simulink model "Relu_OutFB_4_4_1_HW_C6"  (R2012b)
settings: Solver=ode45  StartTime=0.0  StopTime=10.0  RelTol=1e-3
undefined symbols (not defined in the file): alpha, delayMulx, delayMuly, delayROMSig, M2, M3, mu, ts
libraries: xbsIndex_r4 x1583, roblocks x1
(part 3 of 13)

== system Relu_OutFB_4_4_1_HW_C6/EN_MLP_BK_(1,4_NL,1_L)_HW_FPGA/MLP_BK_(2,4_NL,1_L)_HW_FPGA/BK (2,4_NL,1_L)/Subsystem1 ==
  z_1(n) : Inport
  Wy_11(n) : Inport  Port=2
  Gy_11(n) : Inport  Port=3
  Constant : xbsIndex_r4/Constant  const=0  gui_display_data_type=Fixed-point  arith_type=Signed (2's comp)  n_bits=nb  bin_pt=bp  preci_type=Single  exp_width=8  frac_width=24  explicit_period=off  period=1  equ=P=C  opselect=C  inp2=PCIN>>17  opr=+  inp1=P  carry=CIN  dbl_ovrd=off  block_type=constant
  Reinterpret : xbsIndex_r4/Reinterpret  force_arith_type=on  arith_type="Signed  (2's comp)"  force_bin_pt=on  bin_pt=0  block_type=reinterpret
  Relational : xbsIndex_r4/Relational  mode=a<=b  en=off  latency=0  dbl_ovrd=off  block_type=relational
  w_ij(n)*Gy(n) : xbsIndex_r4/Mult  precision=User Defined  arith_type="Signed  (2's comp)"  n_bits=nb  bin_pt=bp  quantization="Round  (unbiased: +/- Inf)"  overflow=Saturate  en=off  latency=delayMuly  dbl_ovrd=off  use_behavioral_HDL=off  opt=Speed  use_embedded=on  optimum_pipeline=off  pipeline=on  use_rpm=on  placement_style=Triangular  block_type=mult
  w_ij(n)*Gy(n)1 : xbsIndex_r4/Mult  precision=User Defined  arith_type="Signed  (2's comp)"  n_bits=nb  bin_pt=bp  quantization="Round  (unbiased: +/- Inf)"  overflow=Saturate  en=off  latency=delayMuly  dbl_ovrd=off  use_behavioral_HDL=off  opt=Speed  use_embedded=on  optimum_pipeline=off  pipeline=on  use_rpm=on  placement_style=Triangular  block_type=mult
  Gx_1(n) : Outport
  wires:
  w_ij(n)*Gy(n)1/1 -> Gx_1(n)/1
  Relational/1 -> Reinterpret/1
  Gy_11(n)/1 -> w_ij(n)*Gy(n)/2
  w_ij(n)*Gy(n)/1 -> w_ij(n)*Gy(n)1/2
  Wy_11(n)/1 -> w_ij(n)*Gy(n)/1
  Constant/1 -> Relational/2
  z_1(n)/1 -> Relational/1
  Reinterpret/1 -> w_ij(n)*Gy(n)1/1

== system Relu_OutFB_4_4_1_HW_C6/EN_MLP_BK_(1,4_NL,1_L)_HW_FPGA/MLP_BK_(2,4_NL,1_L)_HW_FPGA/BK (2,4_NL,1_L)/Subsystem2 ==
  x_0(n) : Inport
  x_1(n) : Inport  Port=2
  Gx_1(n) : Inport  Port=3
  x_2(n) : Inport  Port=4
  x_3(n) : Inport  Port=5
  x_4(n) : Inport  Port=6
  Subsystem1 : Subsystem
  Subsystem2 : Subsystem
  Subsystem3 : Subsystem
  Subsystem5 : Subsystem
  Subsystem6 : Subsystem
  Wx_21(n) : Outport
  Wx_20(n) : Outport  Port=2
  Wx_22(n) : Outport  Port=3
  Wx_23(n) : Outport  Port=4
  Wx_24(n) : Outport  Port=5
  wires:
  Subsystem3/1(Wx_11(n)) -> Wx_24(n)/1
  x_4(n)/1 -> Subsystem3/2(x_1(n))
  Gx_1(n)/1 -> Subsystem6/1(Gx_1(n)), Subsystem1/1(Gx_1(n)), Subsystem2/1(Gx_1(n)), Subsystem3/1(Gx_1(n)), Subsystem5/1(Gx_1(n))
  Subsystem1/1(Wx_11(n)) -> Wx_22(n)/1
  Subsystem2/1(Wx_11(n)) -> Wx_23(n)/1
  x_2(n)/1 -> Subsystem1/2(x_1(n))
  x_3(n)/1 -> Subsystem2/2(x_1(n))
  x_1(n)/1 -> Subsystem6/2(x_1(n))
  Subsystem6/1(Wx_11(n)) -> Wx_21(n)/1
  x_0(n)/1 -> Subsystem5/2(x_0(n))
  Subsystem5/1(Wx_10(n)) -> Wx_20(n)/1

== system Relu_OutFB_4_4_1_HW_C6/EN_MLP_BK_(1,4_NL,1_L)_HW_FPGA/MLP_BK_(2,4_NL,1_L)_HW_FPGA/BK (2,4_NL,1_L)/Subsystem3 ==
  z_1(n) : Inport
  Wy_11(n) : Inport  Port=2
  Gy_11(n) : Inport  Port=3
  Constant : xbsIndex_r4/Constant  const=0  gui_display_data_type=Fixed-point  arith_type=Signed (2's comp)  n_bits=nb  bin_pt=bp  preci_type=Single  exp_width=8  frac_width=24  explicit_period=off  period=1  equ=P=C  opselect=C  inp2=PCIN>>17  opr=+  inp1=P  carry=CIN  dbl_ovrd=off  block_type=constant
  Reinterpret : xbsIndex_r4/Reinterpret  force_arith_type=on  arith_type="Signed  (2's comp)"  force_bin_pt=on  bin_pt=0  block_type=reinterpret
  Relational : xbsIndex_r4/Relational  mode=a<=b  en=off  latency=0  dbl_ovrd=off  block_type=relational
  w_ij(n)*Gy(n) : xbsIndex_r4/Mult  precision=User Defined  arith_type="Signed  (2's comp)"  n_bits=nb  bin_pt=bp  quantization="Round  (unbiased: +/- Inf)"  overflow=Saturate  en=off  latency=delayMuly  dbl_ovrd=off  use_behavioral_HDL=off  opt=Speed  use_embedded=on  optimum_pipeline=off  pipeline=on  use_rpm=on  placement_style=Triangular  block_type=mult
  w_ij(n)*Gy(n)1 : xbsIndex_r4/Mult  precision=User Defined  arith_type="Signed  (2's comp)"  n_bits=nb  bin_pt=bp  quantization="Round  (unbiased: +/- Inf)"  overflow=Saturate  en=off  latency=delayMuly  dbl_ovrd=off  use_behavioral_HDL=off  opt=Speed  use_embedded=on  optimum_pipeline=off  pipeline=on  use_rpm=on  placement_style=Triangular  block_type=mult
  Gx_1(n) : Outport
  wires:
  w_ij(n)*Gy(n)1/1 -> Gx_1(n)/1
  Relational/1 -> Reinterpret/1
  Gy_11(n)/1 -> w_ij(n)*Gy(n)/2
  w_ij(n)*Gy(n)/1 -> w_ij(n)*Gy(n)1/2
  Wy_11(n)/1 -> w_ij(n)*Gy(n)/1
  Constant/1 -> Relational/2
  z_1(n)/1 -> Relational/1
  Reinterpret/1 -> w_ij(n)*Gy(n)1/1

== system Relu_OutFB_4_4_1_HW_C6/EN_MLP_BK_(1,4_NL,1_L)_HW_FPGA/MLP_BK_(2,4_NL,1_L)_HW_FPGA/BK (2,4_NL,1_L)/Subsystem4 ==
  z_1(n) : Inport
  Wy_11(n) : Inport  Port=2
  Gy_11(n) : Inport  Port=3
  Constant : xbsIndex_r4/Constant  const=0  gui_display_data_type=Fixed-point  arith_type=Signed (2's comp)  n_bits=nb  bin_pt=bp  preci_type=Single  exp_width=8  frac_width=24  explicit_period=off  period=1  equ=P=C  opselect=C  inp2=PCIN>>17  opr=+  inp1=P  carry=CIN  dbl_ovrd=off  block_type=constant
  Reinterpret : xbsIndex_r4/Reinterpret  force_arith_type=on  arith_type="Signed  (2's comp)"  force_bin_pt=on  bin_pt=0  block_type=reinterpret
  Relational : xbsIndex_r4/Relational  mode=a<=b  en=off  latency=0  dbl_ovrd=off  block_type=relational
  w_ij(n)*Gy(n) : xbsIndex_r4/Mult  precision=User Defined  arith_type="Signed  (2's comp)"  n_bits=nb  bin_pt=bp  quantization="Round  (unbiased: +/- Inf)"  overflow=Saturate  en=off  latency=delayMuly  dbl_ovrd=off  use_behavioral_HDL=off  opt=Speed  use_embedded=on  optimum_pipeline=off  pipeline=on  use_rpm=on  placement_style=Triangular  block_type=mult
  w_ij(n)*Gy(n)1 : xbsIndex_r4/Mult  precision=User Defined  arith_type="Signed  (2's comp)"  n_bits=nb  bin_pt=bp  quantization="Round  (unbiased: +/- Inf)"  overflow=Saturate  en=off  latency=delayMuly  dbl_ovrd=off  use_behavioral_HDL=off  opt=Speed  use_embedded=on  optimum_pipeline=off  pipeline=on  use_rpm=on  placement_style=Triangular  block_type=mult
  Gx_1(n) : Outport
  wires:
  w_ij(n)*Gy(n)1/1 -> Gx_1(n)/1
  Relational/1 -> Reinterpret/1
  Gy_11(n)/1 -> w_ij(n)*Gy(n)/2
  w_ij(n)*Gy(n)/1 -> w_ij(n)*Gy(n)1/2
  Wy_11(n)/1 -> w_ij(n)*Gy(n)/1
  Constant/1 -> Relational/2
  z_1(n)/1 -> Relational/1
  Reinterpret/1 -> w_ij(n)*Gy(n)1/1

== system Relu_OutFB_4_4_1_HW_C6/EN_MLP_BK_(1,4_NL,1_L)_HW_FPGA/MLP_BK_(2,4_NL,1_L)_HW_FPGA/BK (2,4_NL,1_L)/Subsystem5 ==
  x_0(n) : Inport
  x_1(n) : Inport  Port=2
  Gx_1(n) : Inport  Port=3
  x_2(n) : Inport  Port=4
  x_3(n) : Inport  Port=5
  x_4(n) : Inport  Port=6
  Subsystem1 : Subsystem
  Subsystem2 : Subsystem
  Subsystem3 : Subsystem
  Subsystem5 : Subsystem
  Subsystem6 : Subsystem
  Wx_31(n) : Outport
  Wx_30(n) : Outport  Port=2
  Wx_32(n) : Outport  Port=3
  Wx_33(n) : Outport  Port=4
  Wx_34(n) : Outport  Port=5
  wires:
  Subsystem5/1(Wx_10(n)) -> Wx_30(n)/1
  x_0(n)/1 -> Subsystem5/2(x_0(n))
  Subsystem6/1(Wx_11(n)) -> Wx_31(n)/1
  x_1(n)/1 -> Subsystem6/2(x_1(n))
  x_3(n)/1 -> Subsystem2/2(x_1(n))
  x_2(n)/1 -> Subsystem1/2(x_1(n))
  Subsystem2/1(Wx_11(n)) -> Wx_33(n)/1
  Subsystem1/1(Wx_11(n)) -> Wx_32(n)/1
  Gx_1(n)/1 -> Subsystem5/1(Gx_1(n)), Subsystem3/1(Gx_1(n)), Subsystem2/1(Gx_1(n)), Subsystem1/1(Gx_1(n)), Subsystem6/1(Gx_1(n))
  x_4(n)/1 -> Subsystem3/2(x_1(n))
  Subsystem3/1(Wx_11(n)) -> Wx_34(n)/1

== system Relu_OutFB_4_4_1_HW_C6/EN_MLP_BK_(1,4_NL,1_L)_HW_FPGA/MLP_BK_(2,4_NL,1_L)_HW_FPGA/BK (2,4_NL,1_L)/Subsystem6 ==
  x_0(n) : Inport
  x_1(n) : Inport  Port=2
  Gx_1(n) : Inport  Port=3
  x_2(n) : Inport  Port=4
  x_3(n) : Inport  Port=5
  x_4(n) : Inport  Port=6
  Subsystem1 : Subsystem
  Subsystem2 : Subsystem
  Subsystem3 : Subsystem
  Subsystem5 : Subsystem
  Subsystem6 : Subsystem
  Wx_41(n) : Outport
  Wx_40(n) : Outport  Port=2
  Wx_42(n) : Outport  Port=3
  Wx_43(n) : Outport  Port=4
  Wx_44(n) : Outport  Port=5
  wires:
  Subsystem3/1(Wx_11(n)) -> Wx_44(n)/1
  x_4(n)/1 -> Subsystem3/2(x_1(n))
  Gx_1(n)/1 -> Subsystem6/1(Gx_1(n)), Subsystem1/1(Gx_1(n)), Subsystem2/1(Gx_1(n)), Subsystem3/1(Gx_1(n)), Subsystem5/1(Gx_1(n))
  Subsystem1/1(Wx_11(n)) -> Wx_42(n)/1
  Subsystem2/1(Wx_11(n)) -> Wx_43(n)/1
  x_2(n)/1 -> Subsystem1/2(x_1(n))
  x_3(n)/1 -> Subsystem2/2(x_1(n))
  x_1(n)/1 -> Subsystem6/2(x_1(n))
  Subsystem6/1(Wx_11(n)) -> Wx_41(n)/1
  x_0(n)/1 -> Subsystem5/2(x_0(n))
  Subsystem5/1(Wx_10(n)) -> Wx_40(n)/1

== system Relu_OutFB_4_4_1_HW_C6/EN_MLP_BK_(1,4_NL,1_L)_HW_FPGA/MLP_BK_(2,4_NL,1_L)_HW_FPGA/BK (2,4_NL,1_L)/Subsystem7 ==
  z_1(n) : Inport
  Wy_11(n) : Inport  Port=2
  Gy_11(n) : Inport  Port=3
  Constant : xbsIndex_r4/Constant  const=0  gui_display_data_type=Fixed-point  arith_type=Signed (2's comp)  n_bits=nb  bin_pt=bp  preci_type=Single  exp_width=8  frac_width=24  explicit_period=off  period=1  equ=P=C  opselect=C  inp2=PCIN>>17  opr=+  inp1=P  carry=CIN  dbl_ovrd=off  block_type=constant
  Reinterpret : xbsIndex_r4/Reinterpret  force_arith_type=on  arith_type="Signed  (2's comp)"  force_bin_pt=on  bin_pt=0  block_type=reinterpret
  Relational : xbsIndex_r4/Relational  mode=a<=b  en=off  latency=0  dbl_ovrd=off  block_type=relational
  w_ij(n)*Gy(n) : xbsIndex_r4/Mult  precision=User Defined  arith_type="Signed  (2's comp)"  n_bits=nb  bin_pt=bp  quantization="Round  (unbiased: +/- Inf)"  overflow=Saturate  en=off  latency=delayMuly  dbl_ovrd=off  use_behavioral_HDL=off  opt=Speed  use_embedded=on  optimum_pipeline=off  pipeline=on  use_rpm=on  placement_style=Triangular  block_type=mult
  w_ij(n)*Gy(n)1 : xbsIndex_r4/Mult  precision=User Defined  arith_type="Signed  (2's comp)"  n_bits=nb  bin_pt=bp  quantization="Round  (unbiased: +/- Inf)"  overflow=Saturate  en=off  latency=delayMuly  dbl_ovrd=off  use_behavioral_HDL=off  opt=Speed  use_embedded=on  optimum_pipeline=off  pipeline=on  use_rpm=on  placement_style=Triangular  block_type=mult
  Gx_1(n) : Outport
  wires:
  w_ij(n)*Gy(n)1/1 -> Gx_1(n)/1
  Relational/1 -> Reinterpret/1
  Gy_11(n)/1 -> w_ij(n)*Gy(n)/2
  w_ij(n)*Gy(n)/1 -> w_ij(n)*Gy(n)1/2
  Wy_11(n)/1 -> w_ij(n)*Gy(n)/1
  Constant/1 -> Relational/2
  z_1(n)/1 -> Relational/1
  Reinterpret/1 -> w_ij(n)*Gy(n)1/1

== system Relu_OutFB_4_4_1_HW_C6/EN_MLP_BK_(1,4_NL,1_L)_HW_FPGA/MLP_BK_(2,4_NL,1_L)_HW_FPGA/BK (2,4_NL,1_L)/Subsystem8 ==
  x_0(n) : Inport
  x_1(n) : Inport  Port=2
  Gx_1(n) : Inport  Port=3
  x_2(n) : Inport  Port=4
  x_3(n) : Inport  Port=5
  x_4(n) : Inport  Port=6
  Subsystem1 : Subsystem
  Subsystem2 : Subsystem
  Subsystem3 : Subsystem
  Subsystem5 : Subsystem
  Subsystem6 : Subsystem
  Wx_11(n) : Outport
  Wx_10(n) : Outport  Port=2
  Wx_12(n) : Outport  Port=3
  Wx_13(n) : Outport  Port=4
  Wx_14(n) : Outport  Port=5
  wires:
  Subsystem5/1(Wx_10(n)) -> Wx_10(n)/1
  x_0(n)/1 -> Subsystem5/2(x_0(n))
  Subsystem6/1(Wx_11(n)) -> Wx_11(n)/1
  x_1(n)/1 -> Subsystem6/2(x_1(n))
  x_3(n)/1 -> Subsystem2/2(x_1(n))
  x_2(n)/1 -> Subsystem1/2(x_1(n))
  Subsystem2/1(Wx_13(n)) -> Wx_13(n)/1
  Subsystem1/1(Wx_12(n)) -> Wx_12(n)/1
  Gx_1(n)/1 -> Subsystem5/1(Gx_1(n)), Subsystem3/1(Gx_1(n)), Subsystem2/1(Gx_1(n)), Subsystem1/1(Gx_1(n)), Subsystem6/1(Gx_1(n))
  x_4(n)/1 -> Subsystem3/2(x_1(n))
  Subsystem3/1(Wx_14(n)) -> Wx_14(n)/1

== system Relu_OutFB_4_4_1_HW_C6/EN_MLP_BK_(1,4_NL,1_L)_HW_FPGA/MLP_BK_(2,4_NL,1_L)_HW_FPGA/MLP (2,4_NL,1_L)/Neurônio Linear_HW2 ==
  note: x_p
  note: x_p
  note: x_p
  note: x_p
  note: x_p
  z_0(n) : Inport
  z_1(n) : Inport  Port=2
  z_2(n)1 : Inport  Port=3
  z_3(n)2 : Inport  Port=4
  z_4(n)3 : Inport  Port=5
  w_ij(n)4 : Inport  Port=6
  w_ij(n) : Inport  Port=7
  w_ij(n)1 : Inport  Port=8
  w_ij(n)2 : Inport  Port=9
  w_ij(n)3 : Inport  Port=10
  AddSub{,1..3} (4 alike) : xbsIndex_r4/AddSub  mode=Addition  use_carryin=off  use_carryout=off  en=off  latency=0  precision=User Defined  arith_type="Signed  (2's comp)"  n_bits=nb  bin_pt=bp  quantization="Round  (unbiased: +/- Inf)"  overflow=Wrap  dbl_ovrd=off  use_behavioral_HDL=off  hw_selection=Fabric  pipelined=off  block_type=addsub
  x_p*w_ij(n){,1..4} (5 alike) : xbsIndex_r4/Mult  precision=User Defined  arith_type="Signed  (2's comp)"  n_bits=nb  bin_pt=bp  quantization="Round  (unbiased: +/- Inf)"  overflow=Saturate  en=off  latency=delayMuly  dbl_ovrd=off  use_behavioral_HDL=off  opt=Speed  use_embedded=on  optimum_pipeline=off  pipeline=on  use_rpm=on  placement_style=Triangular  block_type=mult
  y_0(n) : Outport
  wires:
  AddSub2/1 -> AddSub3/2
  w_ij(n)4/1 -> x_p*w_ij(n)4/1  "w_ij(n)"
  z_0(n)/1 -> x_p*w_ij(n)4/2
  x_p*w_ij(n)4/1 -> AddSub3/1  "y_k"
  AddSub1/1 -> AddSub2/2
  AddSub/1 -> AddSub2/1
  w_ij(n)2/1 -> x_p*w_ij(n)2/1  "w_ij(n)"
  z_3(n)2/1 -> x_p*w_ij(n)2/2
  x_p*w_ij(n)2/1 -> AddSub1/1  "y_k"
  w_ij(n)3/1 -> x_p*w_ij(n)3/1  "w_ij(n)"
  z_4(n)3/1 -> x_p*w_ij(n)3/2
  x_p*w_ij(n)3/1 -> AddSub1/2
  w_ij(n)/1 -> x_p*w_ij(n)/1  "w_ij(n)"
  z_1(n)/1 -> x_p*w_ij(n)/2
  x_p*w_ij(n)/1 -> AddSub/1  "y_k"
  w_ij(n)1/1 -> x_p*w_ij(n)1/1  "w_ij(n)"
  z_2(n)1/1 -> x_p*w_ij(n)1/2
  x_p*w_ij(n)1/1 -> AddSub/2
  AddSub3/1 -> y_0(n)/1

== system Relu_OutFB_4_4_1_HW_C6/EN_MLP_BK_(1,4_NL,1_L)_HW_FPGA/MLP_BK_(2,4_NL,1_L)_HW_FPGA/MLP (2,4_NL,1_L)/Neurônio Não-Linear_HW1 ==
  note: x_p
  note: x_p
  x_0(n) : Inport
  x_1(n) : Inport  Port=2
  x_2(n) : Inport  Port=3
  x_3(n) : Inport  Port=4
  x_4(n) : Inport  Port=5
  Wx_20(n) : Inport  Port=6
  Wx_21(n) : Inport  Port=7
  Wx_22(n) : Inport  Port=8
  Wx_23(n) : Inport  Port=9
  Wx_24(n) : Inport  Port=10
  AddSub{1..4} (4 alike) : xbsIndex_r4/AddSub  mode=Addition  use_carryin=off  use_carryout=off  en=off  latency=0  precision=User Defined  arith_type="Signed  (2's comp)"  n_bits=nb  bin_pt=bp  quantization="Round  (unbiased: +/- Inf)"  overflow=Wrap  dbl_ovrd=off  use_behavioral_HDL=off  hw_selection=Fabric  pipelined=off  block_type=addsub
  Subsystem : Subsystem
  x_p*w_ij(n){,1..4} (5 alike) : xbsIndex_r4/Mult  precision=User Defined  arith_type="Signed  (2's comp)"  n_bits=nb  bin_pt=bp  quantization="Round  (unbiased: +/- Inf)"  overflow=Saturate  en=off  latency=delayMulx  dbl_ovrd=off  use_behavioral_HDL=off  opt=Speed  use_embedded=on  optimum_pipeline=off  pipeline=on  use_rpm=on  placement_style=Triangular  block_type=mult
  z_k(n) : Outport
  wires:
  Wx_21(n)/1 -> x_p*w_ij(n)/1  "w_ij(n)"
  x_1(n)/1 -> x_p*w_ij(n)/2
  x_p*w_ij(n)/1 -> AddSub1/2  "y_k"
  Subsystem/1(Out1) -> z_k(n)/1
  Wx_20(n)/1 -> x_p*w_ij(n)2/1  "w_ij(n)"
  x_0(n)/1 -> x_p*w_ij(n)2/2
  x_p*w_ij(n)2/1 -> AddSub1/1
  x_2(n)/1 -> x_p*w_ij(n)1/2
  x_3(n)/1 -> x_p*w_ij(n)3/2
  x_4(n)/1 -> x_p*w_ij(n)4/2
  Wx_22(n)/1 -> x_p*w_ij(n)1/1
  Wx_23(n)/1 -> x_p*w_ij(n)3/1
  Wx_24(n)/1 -> x_p*w_ij(n)4/1
  x_p*w_ij(n)1/1 -> AddSub2/1
  x_p*w_ij(n)3/1 -> AddSub2/2
  x_p*w_ij(n)4/1 -> AddSub3/2
  AddSub2/1 -> AddSub3/1
  AddSub4/1 -> Subsystem/1(In1)
  AddSub3/1 -> AddSub4/2
  AddSub1/1 -> AddSub4/1

== system Relu_OutFB_4_4_1_HW_C6/EN_MLP_BK_(1,4_NL,1_L)_HW_FPGA/MLP_BK_(2,4_NL,1_L)_HW_FPGA/MLP (2,4_NL,1_L)/Neurônio Não-Linear_HW2 ==
  note: x_p
  note: x_p
  x_0(n) : Inport
  x_1(n) : Inport  Port=2
  x_2(n) : Inport  Port=3
  x_3(n) : Inport  Port=4
  x_4(n) : Inport  Port=5
  Wx_10(n) : Inport  Port=6
  Wx_11(n) : Inport  Port=7
  Wx_12(n) : Inport  Port=8
  Wx_13(n) : Inport  Port=9
  Wx_14(n) : Inport  Port=10
  AddSub{1..4} (4 alike) : xbsIndex_r4/AddSub  mode=Addition  use_carryin=off  use_carryout=off  en=off  latency=0  precision=User Defined  arith_type="Signed  (2's comp)"  n_bits=nb  bin_pt=bp  quantization="Round  (unbiased: +/- Inf)"  overflow=Wrap  dbl_ovrd=off  use_behavioral_HDL=off  hw_selection=Fabric  pipelined=off  block_type=addsub
  Subsystem : Subsystem
  x_p*w_ij(n){,1..4} (5 alike) : xbsIndex_r4/Mult  precision=User Defined  arith_type="Signed  (2's comp)"  n_bits=nb  bin_pt=bp  quantization="Round  (unbiased: +/- Inf)"  overflow=Saturate  en=off  latency=delayMulx  dbl_ovrd=off  use_behavioral_HDL=off  opt=Speed  use_embedded=on  optimum_pipeline=off  pipeline=on  use_rpm=on  placement_style=Triangular  block_type=mult
  z_k(n) : Outport
  wires:
  AddSub1/1 -> AddSub4/1
  AddSub4/1 -> Subsystem/1(In1)
  AddSub2/1 -> AddSub3/1
  x_p*w_ij(n)4/1 -> AddSub3/2
  x_p*w_ij(n)3/1 -> AddSub2/2
  x_p*w_ij(n)1/1 -> AddSub2/1
  Wx_14(n)/1 -> x_p*w_ij(n)4/1
  Wx_13(n)/1 -> x_p*w_ij(n)3/1
  Wx_12(n)/1 -> x_p*w_ij(n)1/1
  x_4(n)/1 -> x_p*w_ij(n)4/2
  x_3(n)/1 -> x_p*w_ij(n)3/2
  x_2(n)/1 -> x_p*w_ij(n)1/2
  x_p*w_ij(n)2/1 -> AddSub1/1
  x_0(n)/1 -> x_p*w_ij(n)2/2
  Wx_10(n)/1 -> x_p*w_ij(n)2/1  "w_ij(n)"
  Subsystem/1(Out1) -> z_k(n)/1
  x_p*w_ij(n)/1 -> AddSub1/2  "y_k"
  x_1(n)/1 -> x_p*w_ij(n)/2
  Wx_11(n)/1 -> x_p*w_ij(n)/1  "w_ij(n)"
  AddSub3/1 -> AddSub4/2

== system Relu_OutFB_4_4_1_HW_C6/EN_MLP_BK_(1,4_NL,1_L)_HW_FPGA/MLP_BK_(2,4_NL,1_L)_HW_FPGA/MLP (2,4_NL,1_L)/Neurônio Não-Linear_HW3 ==
  note: x_p
  note: x_p
  x_0(n) : Inport
  x_1(n) : Inport  Port=2
  x_2(n) : Inport  Port=3
  x_3(n) : Inport  Port=4
  x_4(n) : Inport  Port=5
  Wx_30(n) : Inport  Port=6
  Wx_31(n) : Inport  Port=7
  Wx_32(n) : Inport  Port=8
  Wx_33(n) : Inport  Port=9
  Wx_34(n) : Inport  Port=10
  AddSub{1..4} (4 alike) : xbsIndex_r4/AddSub  mode=Addition  use_carryin=off  use_carryout=off  en=off  latency=0  precision=User Defined  arith_type="Signed  (2's comp)"  n_bits=nb  bin_pt=bp  quantization="Round  (unbiased: +/- Inf)"  overflow=Wrap  dbl_ovrd=off  use_behavioral_HDL=off  hw_selection=Fabric  pipelined=off  block_type=addsub
  Subsystem : Subsystem
  x_p*w_ij(n){,1..4} (5 alike) : xbsIndex_r4/Mult  precision=User Defined  arith_type="Signed  (2's comp)"  n_bits=nb  bin_pt=bp  quantization="Round  (unbiased: +/- Inf)"  overflow=Saturate  en=off  latency=delayMulx  dbl_ovrd=off  use_behavioral_HDL=off  opt=Speed  use_embedded=on  optimum_pipeline=off  pipeline=on  use_rpm=on  placement_style=Triangular  block_type=mult
  z_k(n) : Outport
  wires:
  AddSub1/1 -> AddSub4/1
  AddSub3/1 -> AddSub4/2
  AddSub4/1 -> Subsystem/1(In1)
  AddSub2/1 -> AddSub3/1
  x_p*w_ij(n)4/1 -> AddSub3/2
  x_p*w_ij(n)3/1 -> AddSub2/2
  x_p*w_ij(n)1/1 -> AddSub2/1
  Wx_34(n)/1 -> x_p*w_ij(n)4/1
  Wx_33(n)/1 -> x_p*w_ij(n)3/1
  Wx_32(n)/1 -> x_p*w_ij(n)1/1
  x_4(n)/1 -> x_p*w_ij(n)4/2
  x_3(n)/1 -> x_p*w_ij(n)3/2
  x_2(n)/1 -> x_p*w_ij(n)1/2
  x_p*w_ij(n)2/1 -> AddSub1/1
  x_0(n)/1 -> x_p*w_ij(n)2/2
  Wx_30(n)/1 -> x_p*w_ij(n)2/1  "w_ij(n)"
  Subsystem/1(Out1) -> z_k(n)/1
  x_p*w_ij(n)/1 -> AddSub1/2  "y_k"
  x_1(n)/1 -> x_p*w_ij(n)/2
  Wx_31(n)/1 -> x_p*w_ij(n)/1  "w_ij(n)"

== system Relu_OutFB_4_4_1_HW_C6/EN_MLP_BK_(1,4_NL,1_L)_HW_FPGA/MLP_BK_(2,4_NL,1_L)_HW_FPGA/MLP (2,4_NL,1_L)/Neurônio Não-Linear_HW4 ==
  note: x_p
  note: x_p
  x_0(n) : Inport
  x_1(n) : Inport  Port=2
  x_2(n) : Inport  Port=3
  x_3(n) : Inport  Port=4
  x_4(n) : Inport  Port=5
  Wx_40(n) : Inport  Port=6
  Wx_41(n) : Inport  Port=7
  Wx_42(n) : Inport  Port=8
  Wx_43(n) : Inport  Port=9
  Wx_44(n) : Inport  Port=10
  AddSub{1..4} (4 alike) : xbsIndex_r4/AddSub  mode=Addition  use_carryin=off  use_carryout=off  en=off  latency=0  precision=User Defined  arith_type="Signed  (2's comp)"  n_bits=nb  bin_pt=bp  quantization="Round  (unbiased: +/- Inf)"  overflow=Wrap  dbl_ovrd=off  use_behavioral_HDL=off  hw_selection=Fabric  pipelined=off  block_type=addsub
  Subsystem : Subsystem
  x_p*w_ij(n){,1..4} (5 alike) : xbsIndex_r4/Mult  precision=User Defined  arith_type="Signed  (2's comp)"  n_bits=nb  bin_pt=bp  quantization="Round  (unbiased: +/- Inf)"  overflow=Saturate  en=off  latency=delayMulx  dbl_ovrd=off  use_behavioral_HDL=off  opt=Speed  use_embedded=on  optimum_pipeline=off  pipeline=on  use_rpm=on  placement_style=Triangular  block_type=mult
  z_k(n) : Outport
  wires:
  Wx_41(n)/1 -> x_p*w_ij(n)/1  "w_ij(n)"
  x_1(n)/1 -> x_p*w_ij(n)/2
  x_p*w_ij(n)/1 -> AddSub1/2  "y_k"
  Subsystem/1(Out1) -> z_k(n)/1
  Wx_40(n)/1 -> x_p*w_ij(n)2/1  "w_ij(n)"
  x_0(n)/1 -> x_p*w_ij(n)2/2
  x_p*w_ij(n)2/1 -> AddSub1/1
  x_2(n)/1 -> x_p*w_ij(n)1/2
  x_3(n)/1 -> x_p*w_ij(n)3/2
  x_4(n)/1 -> x_p*w_ij(n)4/2
  Wx_42(n)/1 -> x_p*w_ij(n)1/1
  Wx_43(n)/1 -> x_p*w_ij(n)3/1
  Wx_44(n)/1 -> x_p*w_ij(n)4/1
  x_p*w_ij(n)1/1 -> AddSub2/1
  x_p*w_ij(n)3/1 -> AddSub2/2
  x_p*w_ij(n)4/1 -> AddSub3/2
  AddSub2/1 -> AddSub3/1
  AddSub4/1 -> Subsystem/1(In1)
  AddSub3/1 -> AddSub4/2
  AddSub1/1 -> AddSub4/1

== system Relu_OutFB_4_4_1_HW_C6/EN_MLP_BK_(1,4_NL,1_L)_HW_FPGA1/MLP_BK_(2,4_NL,1_L)_HW_FPGA/BK (2,4_NL,1_L)/Camada de Saída0 ==
  z_0(n) : Inport
  e(n) : Inport  Port=2
  AddSub1 : xbsIndex_r4/AddSub  mode=Addition  use_carryin=off  use_carryout=off  en=off  latency=0  precision=User Defined  arith_type="Signed  (2's comp)"  n_bits=nb  bin_pt=bp  quantization=Truncate  overflow=Wrap  dbl_ovrd=off  use_behavioral_HDL=off  hw_selection=Fabric  pipelined=off  block_type=addsub
  AddSub2 : xbsIndex_r4/AddSub  mode=Addition  use_carryin=off  use_carryout=off  en=off  latency=0  precision=User Defined  arith_type="Signed  (2's comp)"  n_bits=nb  bin_pt=bp  quantization=Truncate  overflow=Wrap  dbl_ovrd=off  use_behavioral_HDL=off  hw_selection=Fabric  pipelined=off  block_type=addsub
  CMult : xbsIndex_r4/CMult  const=mu  gui_display_data_type=Fixed-point  const_n_bits=32  const_bin_pt=32  float_type=Single  exp_bits=8  fraction_bits=24  en=off  latency=0  precision=User Defined  arith_type="Signed  (2's comp)"  n_bits=nb  bin_pt=bp  quantization="Round  (unbiased: +/- Inf)"  overflow=Wrap  dbl_ovrd=off  use_behavioral_HDL=off  mem_type=Distributed RAM  pipeline=off  block_type=cmult
  CMult1 : xbsIndex_r4/CMult  const=alpha  gui_display_data_type=Fixed-point  const_n_bits=32  const_bin_pt=32  float_type=Single  exp_bits=8  fraction_bits=24  en=off  latency=0  precision=User Defined  arith_type="Signed  (2's comp)"  n_bits=nb  bin_pt=bp  quantization="Round  (unbiased: +/- Inf)"  overflow=Wrap  dbl_ovrd=off  use_behavioral_HDL=off  mem_type=Distributed RAM  pipeline=off  block_type=cmult
  Register : xbsIndex_r4/Register  init=real(M2(1))  rst=off  en=off  dbl_ovrd=off  block_type=register
  Register1 : xbsIndex_r4/Register  init=0  rst=off  en=off  dbl_ovrd=off  block_type=register
  z_0(n)*e(n) : xbsIndex_r4/Mult  precision=User Defined  arith_type="Signed  (2's comp)"  n_bits=nb  bin_pt=bp  quantization="Round  (unbiased: +/- Inf)"  overflow=Saturate  en=off  latency=delayMuly  dbl_ovrd=off  use_behavioral_HDL=off  opt=Speed  use_embedded=on  optimum_pipeline=off  pipeline=on  use_rpm=on  placement_style=Triangular  block_type=mult
  Wy_10(n) : Outport
  wires:
  Register/1 -> Register1/1, AddSub2/1, Wy_10(n)/1  "w_ij(n)"
  CMult1/1 -> AddSub1/1  "alpha*w_ij(n-1)"
  Register1/1 -> CMult1/1  "w_ij(n-1)"
  AddSub2/1 -> Register/1  "w_ij(n+1)"
  AddSub1/1 -> AddSub2/2
  z_0(n)/1 -> z_0(n)*e(n)/1
  e(n)/1 -> z_0(n)*e(n)/2
  CMult/1 -> AddSub1/2  "dw(n) = z_0(n)*e(n)*mu"
  z_0(n)*e(n)/1 -> CMult/1

== system Relu_OutFB_4_4_1_HW_C6/EN_MLP_BK_(1,4_NL,1_L)_HW_FPGA1/MLP_BK_(2,4_NL,1_L)_HW_FPGA/BK (2,4_NL,1_L)/Camada de Saída1 ==
  z_1(n) : Inport
  e(n) : Inport  Port=2
  AddSub1 : xbsIndex_r4/AddSub  mode=Addition  use_carryin=off  use_carryout=off  en=off  latency=0  precision=User Defined  arith_type="Signed  (2's comp)"  n_bits=nb  bin_pt=bp  quantization=Truncate  overflow=Wrap  dbl_ovrd=off  use_behavioral_HDL=off  hw_selection=Fabric  pipelined=off  block_type=addsub
  AddSub2 : xbsIndex_r4/AddSub  mode=Addition  use_carryin=off  use_carryout=off  en=off  latency=0  precision=User Defined  arith_type="Signed  (2's comp)"  n_bits=nb  bin_pt=bp  quantization=Truncate  overflow=Wrap  dbl_ovrd=off  use_behavioral_HDL=off  hw_selection=Fabric  pipelined=off  block_type=addsub
  CMult : xbsIndex_r4/CMult  const=mu  gui_display_data_type=Fixed-point  const_n_bits=32  const_bin_pt=32  float_type=Single  exp_bits=8  fraction_bits=24  en=off  latency=0  precision=User Defined  arith_type="Signed  (2's comp)"  n_bits=nb  bin_pt=bp  quantization="Round  (unbiased: +/- Inf)"  overflow=Wrap  dbl_ovrd=off  use_behavioral_HDL=off  mem_type=Distributed RAM  pipeline=off  block_type=cmult
  CMult1 : xbsIndex_r4/CMult  const=alpha  gui_display_data_type=Fixed-point  const_n_bits=32  const_bin_pt=32  float_type=Single  exp_bits=8  fraction_bits=24  en=off  latency=0  precision=User Defined  arith_type="Signed  (2's comp)"  n_bits=nb  bin_pt=bp  quantization="Round  (unbiased: +/- Inf)"  overflow=Wrap  dbl_ovrd=off  use_behavioral_HDL=off  mem_type=Distributed RAM  pipeline=off  block_type=cmult
  Register : xbsIndex_r4/Register  init=real(M2(2))  rst=off  en=off  dbl_ovrd=off  block_type=register
  Register1 : xbsIndex_r4/Register  init=0  rst=off  en=off  dbl_ovrd=off  block_type=register
  z_1(n)*e(n) : xbsIndex_r4/Mult  precision=User Defined  arith_type="Signed  (2's comp)"  n_bits=nb  bin_pt=bp  quantization="Round  (unbiased: +/- Inf)"  overflow=Saturate  en=off  latency=delayMuly  dbl_ovrd=off  use_behavioral_HDL=off  opt=Speed  use_embedded=on  optimum_pipeline=off  pipeline=on  use_rpm=on  placement_style=Triangular  block_type=mult
  Wy_11(n) : Outport
  Gy_11(n) : Outport  Port=2
  wires:
  Register/1 -> Register1/1, AddSub2/1, Wy_11(n)/1  "w_ij(n)"
  CMult1/1 -> AddSub1/1  "alpha*w_ij(n-1)"
  Register1/1 -> CMult1/1  "w_ij(n-1)"
  AddSub2/1 -> Register/1  "w_ij(n+1)"
  AddSub1/1 -> AddSub2/2
  z_1(n)/1 -> z_1(n)*e(n)/1
  e(n)/1 -> Gy_11(n)/1, z_1(n)*e(n)/2
  CMult/1 -> AddSub1/2  "dw(n) = z_0(n)*e(n)*mu"
  z_1(n)*e(n)/1 -> CMult/1

== system Relu_OutFB_4_4_1_HW_C6/EN_MLP_BK_(1,4_NL,1_L)_HW_FPGA1/MLP_BK_(2,4_NL,1_L)_HW_FPGA/BK (2,4_NL,1_L)/Camada de Saída2 ==
  z_1(n) : Inport
  e(n) : Inport  Port=2
  AddSub1 : xbsIndex_r4/AddSub  mode=Addition  use_carryin=off  use_carryout=off  en=off  latency=0  precision=User Defined  arith_type="Signed  (2's comp)"  n_bits=nb  bin_pt=bp  quantization=Truncate  overflow=Wrap  dbl_ovrd=off  use_behavioral_HDL=off  hw_selection=Fabric  pipelined=off  block_type=addsub
  AddSub2 : xbsIndex_r4/AddSub  mode=Addition  use_carryin=off  use_carryout=off  en=off  latency=0  precision=User Defined  arith_type="Signed  (2's comp)"  n_bits=nb  bin_pt=bp  quantization=Truncate  overflow=Wrap  dbl_ovrd=off  use_behavioral_HDL=off  hw_selection=Fabric  pipelined=off  block_type=addsub
  CMult : xbsIndex_r4/CMult  const=mu  gui_display_data_type=Fixed-point  const_n_bits=32  const_bin_pt=32  float_type=Single  exp_bits=8  fraction_bits=24  en=off  latency=0  precision=User Defined  arith_type="Signed  (2's comp)"  n_bits=nb  bin_pt=bp  quantization="Round  (unbiased: +/- Inf)"  overflow=Wrap  dbl_ovrd=off  use_behavioral_HDL=off  mem_type=Distributed RAM  pipeline=off  block_type=cmult
  CMult1 : xbsIndex_r4/CMult  const=alpha  gui_display_data_type=Fixed-point  const_n_bits=32  const_bin_pt=32  float_type=Single  exp_bits=8  fraction_bits=24  en=off  latency=0  precision=User Defined  arith_type="Signed  (2's comp)"  n_bits=nb  bin_pt=bp  quantization="Round  (unbiased: +/- Inf)"  overflow=Wrap  dbl_ovrd=off  use_behavioral_HDL=off  mem_type=Distributed RAM  pipeline=off  block_type=cmult
  Register : xbsIndex_r4/Register  init=real(M2(4))  rst=off  en=off  dbl_ovrd=off  block_type=register
  Register1 : xbsIndex_r4/Register  init=0  rst=off  en=off  dbl_ovrd=off  block_type=register
  z_1(n)*e(n) : xbsIndex_r4/Mult  precision=User Defined  arith_type="Signed  (2's comp)"  n_bits=nb  bin_pt=bp  quantization="Round  (unbiased: +/- Inf)"  overflow=Saturate  en=off  latency=delayMuly  dbl_ovrd=off  use_behavioral_HDL=off  opt=Speed  use_embedded=on  optimum_pipeline=off  pipeline=on  use_rpm=on  placement_style=Triangular  block_type=mult
  Wy_11(n) : Outport
  Gy_11(n) : Outport  Port=2
  wires:
  Register/1 -> Register1/1, AddSub2/1, Wy_11(n)/1  "w_ij(n)"
  CMult1/1 -> AddSub1/1  "alpha*w_ij(n-1)"
  Register1/1 -> CMult1/1  "w_ij(n-1)"
  AddSub2/1 -> Register/1  "w_ij(n+1)"
  AddSub1/1 -> AddSub2/2
  z_1(n)/1 -> z_1(n)*e(n)/1
  e(n)/1 -> Gy_11(n)/1, z_1(n)*e(n)/2
  CMult/1 -> AddSub1/2  "dw(n) = z_0(n)*e(n)*mu"
  z_1(n)*e(n)/1 -> CMult/1

== system Relu_OutFB_4_4_1_HW_C6/EN_MLP_BK_(1,4_NL,1_L)_HW_FPGA1/MLP_BK_(2,4_NL,1_L)_HW_FPGA/BK (2,4_NL,1_L)/Camada de Saída3 ==
  z_1(n) : Inport
  e(n) : Inport  Port=2
  AddSub1 : xbsIndex_r4/AddSub  mode=Addition  use_carryin=off  use_carryout=off  en=off  latency=0  precision=User Defined  arith_type="Signed  (2's comp)"  n_bits=nb  bin_pt=bp  quantization=Truncate  overflow=Wrap  dbl_ovrd=off  use_behavioral_HDL=off  hw_selection=Fabric  pipelined=off  block_type=addsub
  AddSub2 : xbsIndex_r4/AddSub  mode=Addition  use_carryin=off  use_carryout=off  en=off  latency=0  precision=User Defined  arith_type="Signed  (2's comp)"  n_bits=nb  bin_pt=bp  quantization=Truncate  overflow=Wrap  dbl_ovrd=off  use_behavioral_HDL=off  hw_selection=Fabric  pipelined=off  block_type=addsub
  CMult : xbsIndex_r4/CMult  const=mu  gui_display_data_type=Fixed-point  const_n_bits=32  const_bin_pt=32  float_type=Single  exp_bits=8  fraction_bits=24  en=off  latency=0  precision=User Defined  arith_type="Signed  (2's comp)"  n_bits=nb  bin_pt=bp  quantization="Round  (unbiased: +/- Inf)"  overflow=Wrap  dbl_ovrd=off  use_behavioral_HDL=off  mem_type=Distributed RAM  pipeline=off  block_type=cmult
  CMult1 : xbsIndex_r4/CMult  const=alpha  gui_display_data_type=Fixed-point  const_n_bits=32  const_bin_pt=32  float_type=Single  exp_bits=8  fraction_bits=24  en=off  latency=0  precision=User Defined  arith_type="Signed  (2's comp)"  n_bits=nb  bin_pt=bp  quantization="Round  (unbiased: +/- Inf)"  overflow=Wrap  dbl_ovrd=off  use_behavioral_HDL=off  mem_type=Distributed RAM  pipeline=off  block_type=cmult
  Register : xbsIndex_r4/Register  init=real(M2(3))  rst=off  en=off  dbl_ovrd=off  block_type=register
  Register1 : xbsIndex_r4/Register  init=0  rst=off  en=off  dbl_ovrd=off  block_type=register
  z_1(n)*e(n) : xbsIndex_r4/Mult  precision=User Defined  arith_type="Signed  (2's comp)"  n_bits=nb  bin_pt=bp  quantization="Round  (unbiased: +/- Inf)"  overflow=Saturate  en=off  latency=delayMuly  dbl_ovrd=off  use_behavioral_HDL=off  opt=Speed  use_embedded=on  optimum_pipeline=off  pipeline=on  use_rpm=on  placement_style=Triangular  block_type=mult
  Wy_11(n) : Outport
  Gy_11(n) : Outport  Port=2
  wires:
  z_1(n)*e(n)/1 -> CMult/1
  CMult/1 -> AddSub1/2  "dw(n) = z_0(n)*e(n)*mu"
  e(n)/1 -> z_1(n)*e(n)/2, Gy_11(n)/1
  z_1(n)/1 -> z_1(n)*e(n)/1
  AddSub1/1 -> AddSub2/2
  AddSub2/1 -> Register/1  "w_ij(n+1)"
  Register1/1 -> CMult1/1  "w_ij(n-1)"
  CMult1/1 -> AddSub1/1  "alpha*w_ij(n-1)"
  Register/1 -> Wy_11(n)/1, AddSub2/1, Register1/1  "w_ij(n)"

== system Relu_OutFB_4_4_1_HW_C6/EN_MLP_BK_(1,4_NL,1_L)_HW_FPGA1/MLP_BK_(2,4_NL,1_L)_HW_FPGA/BK (2,4_NL,1_L)/Camada de Saída4 ==
  z_1(n) : Inport
  e(n) : Inport  Port=2
  AddSub1 : xbsIndex_r4/AddSub  mode=Addition  use_carryin=off  use_carryout=off  en=off  latency=0  precision=User Defined  arith_type="Signed  (2's comp)"  n_bits=nb  bin_pt=bp  quantization=Truncate  overflow=Wrap  dbl_ovrd=off  use_behavioral_HDL=off  hw_selection=Fabric  pipelined=off  block_type=addsub
  AddSub2 : xbsIndex_r4/AddSub  mode=Addition  use_carryin=off  use_carryout=off  en=off  latency=0  precision=User Defined  arith_type="Signed  (2's comp)"  n_bits=nb  bin_pt=bp  quantization=Truncate  overflow=Wrap  dbl_ovrd=off  use_behavioral_HDL=off  hw_selection=Fabric  pipelined=off  block_type=addsub
  CMult : xbsIndex_r4/CMult  const=mu  gui_display_data_type=Fixed-point  const_n_bits=32  const_bin_pt=32  float_type=Single  exp_bits=8  fraction_bits=24  en=off  latency=0  precision=User Defined  arith_type="Signed  (2's comp)"  n_bits=nb  bin_pt=bp  quantization="Round  (unbiased: +/- Inf)"  overflow=Wrap  dbl_ovrd=off  use_behavioral_HDL=off  mem_type=Distributed RAM  pipeline=off  block_type=cmult
  CMult1 : xbsIndex_r4/CMult  const=alpha  gui_display_data_type=Fixed-point  const_n_bits=32  const_bin_pt=32  float_type=Single  exp_bits=8  fraction_bits=24  en=off  latency=0  precision=User Defined  arith_type="Signed  (2's comp)"  n_bits=nb  bin_pt=bp  quantization="Round  (unbiased: +/- Inf)"  overflow=Wrap  dbl_ovrd=off  use_behavioral_HDL=off  mem_type=Distributed RAM  pipeline=off  block_type=cmult
  Register : xbsIndex_r4/Register  init=real(M2(5))  rst=off  en=off  dbl_ovrd=off  block_type=register
  Register1 : xbsIndex_r4/Register  init=0  rst=off  en=off  dbl_ovrd=off  block_type=register
  z_1(n)*e(n) : xbsIndex_r4/Mult  precision=User Defined  arith_type="Signed  (2's comp)"  n_bits=nb  bin_pt=bp  quantization="Round  (unbiased: +/- Inf)"  overflow=Saturate  en=off  latency=delayMuly  dbl_ovrd=off  use_behavioral_HDL=off  opt=Speed  use_embedded=on  optimum_pipeline=off  pipeline=on  use_rpm=on  placement_style=Triangular  block_type=mult
  Wy_11(n) : Outport
  Gy_11(n) : Outport  Port=2
  wires:
  z_1(n)*e(n)/1 -> CMult/1
  CMult/1 -> AddSub1/2  "dw(n) = z_0(n)*e(n)*mu"
  e(n)/1 -> z_1(n)*e(n)/2, Gy_11(n)/1
  z_1(n)/1 -> z_1(n)*e(n)/1
  AddSub1/1 -> AddSub2/2
  AddSub2/1 -> Register/1  "w_ij(n+1)"
  Register1/1 -> CMult1/1  "w_ij(n-1)"
  CMult1/1 -> AddSub1/1  "alpha*w_ij(n-1)"
  Register/1 -> Wy_11(n)/1, AddSub2/1, Register1/1  "w_ij(n)"

== system Relu_OutFB_4_4_1_HW_C6/EN_MLP_BK_(1,4_NL,1_L)_HW_FPGA1/MLP_BK_(2,4_NL,1_L)_HW_FPGA/BK (2,4_NL,1_L)/Subsystem1 ==
  z_1(n) : Inport
  Wy_11(n) : Inport  Port=2
  Gy_11(n) : Inport  Port=3
  Constant : xbsIndex_r4/Constant  const=0  gui_display_data_type=Fixed-point  arith_type=Signed (2's comp)  n_bits=nb  bin_pt=bp  preci_type=Single  exp_width=8  frac_width=24  explicit_period=off  period=1  equ=P=C  opselect=C  inp2=PCIN>>17  opr=+  inp1=P  carry=CIN  dbl_ovrd=off  block_type=constant
  Reinterpret : xbsIndex_r4/Reinterpret  force_arith_type=on  arith_type="Signed  (2's comp)"  force_bin_pt=on  bin_pt=0  block_type=reinterpret
  Relational : xbsIndex_r4/Relational  mode=a<=b  en=off  latency=0  dbl_ovrd=off  block_type=relational
  w_ij(n)*Gy(n) : xbsIndex_r4/Mult  precision=User Defined  arith_type="Signed  (2's comp)"  n_bits=nb  bin_pt=bp  quantization="Round  (unbiased: +/- Inf)"  overflow=Saturate  en=off  latency=delayMuly  dbl_ovrd=off  use_behavioral_HDL=off  opt=Speed  use_embedded=on  optimum_pipeline=off  pipeline=on  use_rpm=on  placement_style=Triangular  block_type=mult
  w_ij(n)*Gy(n)1 : xbsIndex_r4/Mult  precision=User Defined  arith_type="Signed  (2's comp)"  n_bits=nb  bin_pt=bp  quantization="Round  (unbiased: +/- Inf)"  overflow=Saturate  en=off  latency=delayMuly  dbl_ovrd=off  use_behavioral_HDL=off  opt=Speed  use_embedded=on  optimum_pipeline=off  pipeline=on  use_rpm=on  placement_style=Triangular  block_type=mult
  Gx_1(n) : Outport
  wires:
  w_ij(n)*Gy(n)1/1 -> Gx_1(n)/1
  Relational/1 -> Reinterpret/1
  Gy_11(n)/1 -> w_ij(n)*Gy(n)/2
  w_ij(n)*Gy(n)/1 -> w_ij(n)*Gy(n)1/2
  Wy_11(n)/1 -> w_ij(n)*Gy(n)/1
  Constant/1 -> Relational/2
  z_1(n)/1 -> Relational/1
  Reinterpret/1 -> w_ij(n)*Gy(n)1/1

== system Relu_OutFB_4_4_1_HW_C6/EN_MLP_BK_(1,4_NL,1_L)_HW_FPGA1/MLP_BK_(2,4_NL,1_L)_HW_FPGA/BK (2,4_NL,1_L)/Subsystem2 ==
  x_0(n) : Inport
  x_1(n) : Inport  Port=2
  Gx_1(n) : Inport  Port=3
  x_2(n) : Inport  Port=4
  x_3(n) : Inport  Port=5
  x_4(n) : Inport  Port=6
  Subsystem1 : Subsystem
  Subsystem2 : Subsystem
  Subsystem3 : Subsystem
  Subsystem5 : Subsystem
  Subsystem6 : Subsystem
  Wx_21(n) : Outport
  Wx_20(n) : Outport  Port=2
  Wx_22(n) : Outport  Port=3
  Wx_23(n) : Outport  Port=4
  Wx_24(n) : Outport  Port=5
  wires:
  Subsystem3/1(Wx_11(n)) -> Wx_24(n)/1
  x_4(n)/1 -> Subsystem3/2(x_1(n))
  Gx_1(n)/1 -> Subsystem6/1(Gx_1(n)), Subsystem1/1(Gx_1(n)), Subsystem2/1(Gx_1(n)), Subsystem3/1(Gx_1(n)), Subsystem5/1(Gx_1(n))
  Subsystem1/1(Wx_11(n)) -> Wx_22(n)/1
  Subsystem2/1(Wx_11(n)) -> Wx_23(n)/1
  x_2(n)/1 -> Subsystem1/2(x_1(n))
  x_3(n)/1 -> Subsystem2/2(x_1(n))
  x_1(n)/1 -> Subsystem6/2(x_1(n))
  Subsystem6/1(Wx_11(n)) -> Wx_21(n)/1
  x_0(n)/1 -> Subsystem5/2(x_0(n))
  Subsystem5/1(Wx_10(n)) -> Wx_20(n)/1

== system Relu_OutFB_4_4_1_HW_C6/EN_MLP_BK_(1,4_NL,1_L)_HW_FPGA1/MLP_BK_(2,4_NL,1_L)_HW_FPGA/BK (2,4_NL,1_L)/Subsystem3 ==
  z_1(n) : Inport
  Wy_11(n) : Inport  Port=2
  Gy_11(n) : Inport  Port=3
  Constant : xbsIndex_r4/Constant  const=0  gui_display_data_type=Fixed-point  arith_type=Signed (2's comp)  n_bits=nb  bin_pt=bp  preci_type=Single  exp_width=8  frac_width=24  explicit_period=off  period=1  equ=P=C  opselect=C  inp2=PCIN>>17  opr=+  inp1=P  carry=CIN  dbl_ovrd=off  block_type=constant
  Reinterpret : xbsIndex_r4/Reinterpret  force_arith_type=on  arith_type="Signed  (2's comp)"  force_bin_pt=on  bin_pt=0  block_type=reinterpret
  Relational : xbsIndex_r4/Relational  mode=a<=b  en=off  latency=0  dbl_ovrd=off  block_type=relational
  w_ij(n)*Gy(n) : xbsIndex_r4/Mult  precision=User Defined  arith_type="Signed  (2's comp)"  n_bits=nb  bin_pt=bp  quantization="Round  (unbiased: +/- Inf)"  overflow=Saturate  en=off  latency=delayMuly  dbl_ovrd=off  use_behavioral_HDL=off  opt=Speed  use_embedded=on  optimum_pipeline=off  pipeline=on  use_rpm=on  placement_style=Triangular  block_type=mult
  w_ij(n)*Gy(n)1 : xbsIndex_r4/Mult  precision=User Defined  arith_type="Signed  (2's comp)"  n_bits=nb  bin_pt=bp  quantization="Round  (unbiased: +/- Inf)"  overflow=Saturate  en=off  latency=delayMuly  dbl_ovrd=off  use_behavioral_HDL=off  opt=Speed  use_embedded=on  optimum_pipeline=off  pipeline=on  use_rpm=on  placement_style=Triangular  block_type=mult
  Gx_1(n) : Outport
  wires:
  w_ij(n)*Gy(n)1/1 -> Gx_1(n)/1
  Relational/1 -> Reinterpret/1
  Gy_11(n)/1 -> w_ij(n)*Gy(n)/2
  w_ij(n)*Gy(n)/1 -> w_ij(n)*Gy(n)1/2
  Wy_11(n)/1 -> w_ij(n)*Gy(n)/1
  Constant/1 -> Relational/2
  z_1(n)/1 -> Relational/1
  Reinterpret/1 -> w_ij(n)*Gy(n)1/1

== system Relu_OutFB_4_4_1_HW_C6/EN_MLP_BK_(1,4_NL,1_L)_HW_FPGA1/MLP_BK_(2,4_NL,1_L)_HW_FPGA/BK (2,4_NL,1_L)/Subsystem4 ==
  z_1(n) : Inport
  Wy_11(n) : Inport  Port=2
  Gy_11(n) : Inport  Port=3
  Constant : xbsIndex_r4/Constant  const=0  gui_display_data_type=Fixed-point  arith_type=Signed (2's comp)  n_bits=nb  bin_pt=bp  preci_type=Single  exp_width=8  frac_width=24  explicit_period=off  period=1  equ=P=C  opselect=C  inp2=PCIN>>17  opr=+  inp1=P  carry=CIN  dbl_ovrd=off  block_type=constant
  Reinterpret : xbsIndex_r4/Reinterpret  force_arith_type=on  arith_type="Signed  (2's comp)"  force_bin_pt=on  bin_pt=0  block_type=reinterpret
  Relational : xbsIndex_r4/Relational  mode=a<=b  en=off  latency=0  dbl_ovrd=off  block_type=relational
  w_ij(n)*Gy(n) : xbsIndex_r4/Mult  precision=User Defined  arith_type="Signed  (2's comp)"  n_bits=nb  bin_pt=bp  quantization="Round  (unbiased: +/- Inf)"  overflow=Saturate  en=off  latency=delayMuly  dbl_ovrd=off  use_behavioral_HDL=off  opt=Speed  use_embedded=on  optimum_pipeline=off  pipeline=on  use_rpm=on  placement_style=Triangular  block_type=mult
  w_ij(n)*Gy(n)1 : xbsIndex_r4/Mult  precision=User Defined  arith_type="Signed  (2's comp)"  n_bits=nb  bin_pt=bp  quantization="Round  (unbiased: +/- Inf)"  overflow=Saturate  en=off  latency=delayMuly  dbl_ovrd=off  use_behavioral_HDL=off  opt=Speed  use_embedded=on  optimum_pipeline=off  pipeline=on  use_rpm=on  placement_style=Triangular  block_type=mult
  Gx_1(n) : Outport
  wires:
  w_ij(n)*Gy(n)1/1 -> Gx_1(n)/1
  Relational/1 -> Reinterpret/1
  Gy_11(n)/1 -> w_ij(n)*Gy(n)/2
  w_ij(n)*Gy(n)/1 -> w_ij(n)*Gy(n)1/2
  Wy_11(n)/1 -> w_ij(n)*Gy(n)/1
  Constant/1 -> Relational/2
  z_1(n)/1 -> Relational/1
  Reinterpret/1 -> w_ij(n)*Gy(n)1/1

== system Relu_OutFB_4_4_1_HW_C6/EN_MLP_BK_(1,4_NL,1_L)_HW_FPGA1/MLP_BK_(2,4_NL,1_L)_HW_FPGA/BK (2,4_NL,1_L)/Subsystem5 ==
  x_0(n) : Inport
  x_1(n) : Inport  Port=2
  Gx_1(n) : Inport  Port=3
  x_2(n) : Inport  Port=4
  x_3(n) : Inport  Port=5
  x_4(n) : Inport  Port=6
  Subsystem1 : Subsystem
  Subsystem2 : Subsystem
  Subsystem3 : Subsystem
  Subsystem5 : Subsystem
  Subsystem6 : Subsystem
  Wx_31(n) : Outport
  Wx_30(n) : Outport  Port=2
  Wx_32(n) : Outport  Port=3
  Wx_33(n) : Outport  Port=4
  Wx_34(n) : Outport  Port=5
  wires:
  Subsystem5/1(Wx_10(n)) -> Wx_30(n)/1
  x_0(n)/1 -> Subsystem5/2(x_0(n))
  Subsystem6/1(Wx_11(n)) -> Wx_31(n)/1
  x_1(n)/1 -> Subsystem6/2(x_1(n))
  x_3(n)/1 -> Subsystem2/2(x_1(n))
  x_2(n)/1 -> Subsystem1/2(x_1(n))
  Subsystem2/1(Wx_11(n)) -> Wx_33(n)/1
  Subsystem1/1(Wx_11(n)) -> Wx_32(n)/1
  Gx_1(n)/1 -> Subsystem5/1(Gx_1(n)), Subsystem3/1(Gx_1(n)), Subsystem2/1(Gx_1(n)), Subsystem1/1(Gx_1(n)), Subsystem6/1(Gx_1(n))
  x_4(n)/1 -> Subsystem3/2(x_1(n))
  Subsystem3/1(Wx_11(n)) -> Wx_34(n)/1

== system Relu_OutFB_4_4_1_HW_C6/EN_MLP_BK_(1,4_NL,1_L)_HW_FPGA1/MLP_BK_(2,4_NL,1_L)_HW_FPGA/BK (2,4_NL,1_L)/Subsystem6 ==
  x_0(n) : Inport
  x_1(n) : Inport  Port=2
  Gx_1(n) : Inport  Port=3
  x_2(n) : Inport  Port=4
  x_3(n) : Inport  Port=5
  x_4(n) : Inport  Port=6
  Subsystem1 : Subsystem
  Subsystem2 : Subsystem
  Subsystem3 : Subsystem
  Subsystem5 : Subsystem
  Subsystem6 : Subsystem
  Wx_41(n) : Outport
  Wx_40(n) : Outport  Port=2
  Wx_42(n) : Outport  Port=3
  Wx_43(n) : Outport  Port=4
  Wx_44(n) : Outport  Port=5
  wires:
  Subsystem3/1(Wx_11(n)) -> Wx_44(n)/1
  x_4(n)/1 -> Subsystem3/2(x_1(n))
  Gx_1(n)/1 -> Subsystem6/1(Gx_1(n)), Subsystem1/1(Gx_1(n)), Subsystem2/1(Gx_1(n)), Subsystem3/1(Gx_1(n)), Subsystem5/1(Gx_1(n))
  Subsystem1/1(Wx_11(n)) -> Wx_42(n)/1
  Subsystem2/1(Wx_11(n)) -> Wx_43(n)/1
  x_2(n)/1 -> Subsystem1/2(x_1(n))
  x_3(n)/1 -> Subsystem2/2(x_1(n))
  x_1(n)/1 -> Subsystem6/2(x_1(n))
  Subsystem6/1(Wx_11(n)) -> Wx_41(n)/1
  x_0(n)/1 -> Subsystem5/2(x_0(n))
  Subsystem5/1(Wx_10(n)) -> Wx_40(n)/1

== system Relu_OutFB_4_4_1_HW_C6/EN_MLP_BK_(1,4_NL,1_L)_HW_FPGA1/MLP_BK_(2,4_NL,1_L)_HW_FPGA/BK (2,4_NL,1_L)/Subsystem7 ==
  z_1(n) : Inport
  Wy_11(n) : Inport  Port=2
  Gy_11(n) : Inport  Port=3
  Constant : xbsIndex_r4/Constant  const=0  gui_display_data_type=Fixed-point  arith_type=Signed (2's comp)  n_bits=nb  bin_pt=bp  preci_type=Single  exp_width=8  frac_width=24  explicit_period=off  period=1  equ=P=C  opselect=C  inp2=PCIN>>17  opr=+  inp1=P  carry=CIN  dbl_ovrd=off  block_type=constant
  Reinterpret : xbsIndex_r4/Reinterpret  force_arith_type=on  arith_type="Signed  (2's comp)"  force_bin_pt=on  bin_pt=0  block_type=reinterpret
  Relational : xbsIndex_r4/Relational  mode=a<=b  en=off  latency=0  dbl_ovrd=off  block_type=relational
  w_ij(n)*Gy(n) : xbsIndex_r4/Mult  precision=User Defined  arith_type="Signed  (2's comp)"  n_bits=nb  bin_pt=bp  quantization="Round  (unbiased: +/- Inf)"  overflow=Saturate  en=off  latency=delayMuly  dbl_ovrd=off  use_behavioral_HDL=off  opt=Speed  use_embedded=on  optimum_pipeline=off  pipeline=on  use_rpm=on  placement_style=Triangular  block_type=mult
  w_ij(n)*Gy(n)1 : xbsIndex_r4/Mult  precision=User Defined  arith_type="Signed  (2's comp)"  n_bits=nb  bin_pt=bp  quantization="Round  (unbiased: +/- Inf)"  overflow=Saturate  en=off  latency=delayMuly  dbl_ovrd=off  use_behavioral_HDL=off  opt=Speed  use_embedded=on  optimum_pipeline=off  pipeline=on  use_rpm=on  placement_style=Triangular  block_type=mult
  Gx_1(n) : Outport
  wires:
  w_ij(n)*Gy(n)1/1 -> Gx_1(n)/1
  Relational/1 -> Reinterpret/1
  Gy_11(n)/1 -> w_ij(n)*Gy(n)/2
  w_ij(n)*Gy(n)/1 -> w_ij(n)*Gy(n)1/2
  Wy_11(n)/1 -> w_ij(n)*Gy(n)/1
  Constant/1 -> Relational/2
  z_1(n)/1 -> Relational/1
  Reinterpret/1 -> w_ij(n)*Gy(n)1/1

== system Relu_OutFB_4_4_1_HW_C6/EN_MLP_BK_(1,4_NL,1_L)_HW_FPGA1/MLP_BK_(2,4_NL,1_L)_HW_FPGA/BK (2,4_NL,1_L)/Subsystem8 ==
  x_0(n) : Inport
  x_1(n) : Inport  Port=2
  Gx_1(n) : Inport  Port=3
  x_2(n) : Inport  Port=4
  x_3(n) : Inport  Port=5
  x_4(n) : Inport  Port=6
  Subsystem1 : Subsystem
  Subsystem2 : Subsystem
  Subsystem3 : Subsystem
  Subsystem5 : Subsystem
  Subsystem6 : Subsystem
  Wx_11(n) : Outport
  Wx_10(n) : Outport  Port=2
  Wx_12(n) : Outport  Port=3
  Wx_13(n) : Outport  Port=4
  Wx_14(n) : Outport  Port=5
  wires:
  Subsystem5/1(Wx_10(n)) -> Wx_10(n)/1
  x_0(n)/1 -> Subsystem5/2(x_0(n))
  Subsystem6/1(Wx_11(n)) -> Wx_11(n)/1
  x_1(n)/1 -> Subsystem6/2(x_1(n))
  x_3(n)/1 -> Subsystem2/2(x_1(n))
  x_2(n)/1 -> Subsystem1/2(x_1(n))
  Subsystem2/1(Wx_13(n)) -> Wx_13(n)/1
  Subsystem1/1(Wx_12(n)) -> Wx_12(n)/1
  Gx_1(n)/1 -> Subsystem5/1(Gx_1(n)), Subsystem3/1(Gx_1(n)), Subsystem2/1(Gx_1(n)), Subsystem1/1(Gx_1(n)), Subsystem6/1(Gx_1(n))
  x_4(n)/1 -> Subsystem3/2(x_1(n))
  Subsystem3/1(Wx_14(n)) -> Wx_14(n)/1

== system Relu_OutFB_4_4_1_HW_C6/EN_MLP_BK_(1,4_NL,1_L)_HW_FPGA1/MLP_BK_(2,4_NL,1_L)_HW_FPGA/MLP (2,4_NL,1_L)/Neurônio Linear_HW2 ==
  note: x_p
  note: x_p
  note: x_p
  note: x_p
  note: x_p
  z_0(n) : Inport
  z_1(n) : Inport  Port=2
  z_2(n)1 : Inport  Port=3
  z_3(n)2 : Inport  Port=4
  z_4(n)3 : Inport  Port=5
  w_ij(n)4 : Inport  Port=6
  w_ij(n) : Inport  Port=7
  w_ij(n)1 : Inport  Port=8
  w_ij(n)2 : Inport  Port=9
  w_ij(n)3 : Inport  Port=10
  AddSub{,1..3} (4 alike) : xbsIndex_r4/AddSub  mode=Addition  use_carryin=off  use_carryout=off  en=off  latency=0  precision=User Defined  arith_type="Signed  (2's comp)"  n_bits=nb  bin_pt=bp  quantization="Round  (unbiased: +/- Inf)"  overflow=Wrap  dbl_ovrd=off  use_behavioral_HDL=off  hw_selection=Fabric  pipelined=off  block_type=addsub
  x_p*w_ij(n){,1..4} (5 alike) : xbsIndex_r4/Mult  precision=User Defined  arith_type="Signed  (2's comp)"  n_bits=nb  bin_pt=bp  quantization="Round  (unbiased: +/- Inf)"  overflow=Saturate  en=off  latency=delayMuly  dbl_ovrd=off  use_behavioral_HDL=off  opt=Speed  use_embedded=on  optimum_pipeline=off  pipeline=on  use_rpm=on  placement_style=Triangular  block_type=mult
  y_0(n) : Outport
  wires:
  AddSub2/1 -> AddSub3/2
  w_ij(n)4/1 -> x_p*w_ij(n)4/1  "w_ij(n)"
  z_0(n)/1 -> x_p*w_ij(n)4/2
  x_p*w_ij(n)4/1 -> AddSub3/1  "y_k"
  AddSub1/1 -> AddSub2/2
  AddSub/1 -> AddSub2/1
  w_ij(n)2/1 -> x_p*w_ij(n)2/1  "w_ij(n)"
  z_3(n)2/1 -> x_p*w_ij(n)2/2
  x_p*w_ij(n)2/1 -> AddSub1/1  "y_k"
  w_ij(n)3/1 -> x_p*w_ij(n)3/1  "w_ij(n)"
  z_4(n)3/1 -> x_p*w_ij(n)3/2
  x_p*w_ij(n)3/1 -> AddSub1/2
  w_ij(n)/1 -> x_p*w_ij(n)/1  "w_ij(n)"
  z_1(n)/1 -> x_p*w_ij(n)/2
  x_p*w_ij(n)/1 -> AddSub/1  "y_k"
  w_ij(n)1/1 -> x_p*w_ij(n)1/1  "w_ij(n)"
  z_2(n)1/1 -> x_p*w_ij(n)1/2
  x_p*w_ij(n)1/1 -> AddSub/2
  AddSub3/1 -> y_0(n)/1

== system Relu_OutFB_4_4_1_HW_C6/EN_MLP_BK_(1,4_NL,1_L)_HW_FPGA1/MLP_BK_(2,4_NL,1_L)_HW_FPGA/MLP (2,4_NL,1_L)/Neurônio Não-Linear_HW1 ==
  note: x_p
  note: x_p
  x_0(n) : Inport
  x_1(n) : Inport  Port=2
  x_2(n) : Inport  Port=3
  x_3(n) : Inport  Port=4
  x_4(n) : Inport  Port=5
  Wx_20(n) : Inport  Port=6
  Wx_21(n) : Inport  Port=7
  Wx_22(n) : Inport  Port=8
  Wx_23(n) : Inport  Port=9
  Wx_24(n) : Inport  Port=10
  AddSub{1..4} (4 alike) : xbsIndex_r4/AddSub  mode=Addition  use_carryin=off  use_carryout=off  en=off  latency=0  precision=User Defined  arith_type="Signed  (2's comp)"  n_bits=nb  bin_pt=bp  quantization="Round  (unbiased: +/- Inf)"  overflow=Wrap  dbl_ovrd=off  use_behavioral_HDL=off  hw_selection=Fabric  pipelined=off  block_type=addsub
  Subsystem : Subsystem
  x_p*w_ij(n){,1..4} (5 alike) : xbsIndex_r4/Mult  precision=User Defined  arith_type="Signed  (2's comp)"  n_bits=nb  bin_pt=bp  quantization="Round  (unbiased: +/- Inf)"  overflow=Saturate  en=off  latency=delayMulx  dbl_ovrd=off  use_behavioral_HDL=off  opt=Speed  use_embedded=on  optimum_pipeline=off  pipeline=on  use_rpm=on  placement_style=Triangular  block_type=mult
  z_k(n) : Outport
  wires:
  Wx_21(n)/1 -> x_p*w_ij(n)/1  "w_ij(n)"
  x_1(n)/1 -> x_p*w_ij(n)/2
  x_p*w_ij(n)/1 -> AddSub1/2  "y_k"
  Subsystem/1(Out1) -> z_k(n)/1
  Wx_20(n)/1 -> x_p*w_ij(n)2/1  "w_ij(n)"
  x_0(n)/1 -> x_p*w_ij(n)2/2
  x_p*w_ij(n)2/1 -> AddSub1/1
  x_2(n)/1 -> x_p*w_ij(n)1/2
  x_3(n)/1 -> x_p*w_ij(n)3/2
  x_4(n)/1 -> x_p*w_ij(n)4/2
  Wx_22(n)/1 -> x_p*w_ij(n)1/1
  Wx_23(n)/1 -> x_p*w_ij(n)3/1
  Wx_24(n)/1 -> x_p*w_ij(n)4/1
  x_p*w_ij(n)1/1 -> AddSub2/1
  x_p*w_ij(n)3/1 -> AddSub2/2
  x_p*w_ij(n)4/1 -> AddSub3/2
  AddSub2/1 -> AddSub3/1
  AddSub4/1 -> Subsystem/1(In1)
  AddSub3/1 -> AddSub4/2
  AddSub1/1 -> AddSub4/1
